simulink model "alternatesim1"  (Simulink 9.3)
settings: Solver=FixedStepAuto  StartTime=0.0  StopTime=7  RelTol=1e-3
libraries: neural x1
settings Model: Creator=Lenovo  LastModifiedBy=Lenovo
settings DataIOCC: SaveFormat=Dataset  SignalLoggingSaveFormat=Dataset  ReturnWorkspaceOutputs=on
settings OptimizationCC: LifeSpan=auto
settings DebuggingCC: UnderspecifiedInitializationDetection=Simplified  MergeDetectMultiDrivingBlocksExec=error  FcnCallInpInsideContextMsg=error  SFUnexpectedBacktrackingDiag=error  SFNoUnconditionalDefaultTransitionDiag=error  SFExecutionAtInitializationDiag=warning  ArithmeticOperatorsInVariantConditions=error
settings HardwareCC: ProdBitPerPointer=64  ProdBitPerSizeT=64  ProdBitPerPtrDiffT=64  ProdLargestAtomicFloat=Float  ProdIntDivRoundTo=Zero  ProdEndianess=LittleEndian  ProdWordSize=64  ProdHWDeviceType=Intel->x86-64 (Windows64)
settings ModelReferenceCC: PropagateSignalLabelsOutOfModel=on
settings SFSimCC: SimUseLocalCustomCode=on
settings RTWCC: RTWUseLocalCustomCode=on
settings CodeAppCC: StateflowObjectComments=off
settings GRTTargetCC: TargetLangStandard=C99 (ISO)  CombineOutputUpdateFcns=on  GRTInterface=off
settings ConfigComp: CovMetricSettings=dwe  CovHtmlReporting=off  CovSaveCumulativeToWorkspaceVar=off  CovSaveSingleToWorkspaceVar=off  CovExternalEMLEnable=on

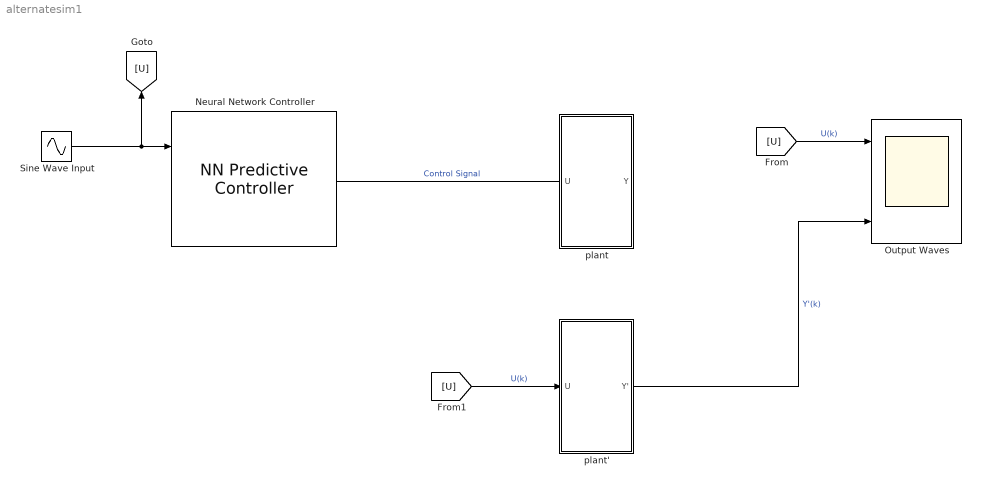
== system alternatesim1 ==
  Neural Network Controller : neural/Control Systems/NN Predictive Controller  epochs=150  minp=-1.4984328739291656873  maxp=1.4972411842840820384  mint=-0.49955219239929099517  maxt=1.4972411842840820384  Normalize=0  IW=[2.1565747230120617672 -0.3096984252732051246;-0.12313821449709881628 -0.1122642020318464634;-0.58041432517589952589 -0.21396504389264983659;0.19499335953396529364 -0.077631398333984871774;0.75410004063625590831 -0.16226526156567477877]  LW1_2=[0.5551207293764637285 0.018714294291257507069;-0.10132675699843593509 -0.027382341482495679841;-0.43309173846840326449 -0.0781007196607201859;-0.3314677820543142639 -0.032004154570293125159;-0.194985926119772085 -0.091076348073804089256]  LW2_1=[1.5809740000360821277 -1.0538130207537415028 -0.24233406046636835063 0.7751203522283688363 0.29703906315315625752]  B1=[-4.5237611134154054326;-0.05295680763842128963;1.2919589532592146153;0.17974555254224580669;-1.0663040710382076792]  B2=1.8293317221646907544  max_i_int=10  min_i_int=2  limit_output=0  max_output=Inf  min_output=-Inf  Use_Previous_Weights=1  N2=10  Nu=2  Ts=0.2  rho=0.05  alpha=0.001  csrchfun=csrchbac  maxiter=2  S1=5  Ni=2  Nj=2  sim_file=plant1  trainfun=trainbr  Use_validation=1  Use_Testing=0  max_i=1.5  min_i=-1.5  sam_training=10000
      settings: SourceProductName=MATLAB Runtime - Deep Learning Toolbox  SourceProductBaseCode=Missing
  Output Waves : Scope  NumInputPorts=3
  Sine Wave Input : Sin  Amplitude=0.8  Frequency=2  SampleTime=0.2
  plant : Subsystem
  plant' : Subsystem
  wires:
  ? -> Neural Network Controller/2, Output Waves/2  "Y(k)"
  Neural Network Controller/1 -> ?  "Control Signal"
  [U] -> Output Waves/1  "U(k)"
  [U] -> plant'/1(U)  "U(k)"
  plant'/1(Y') -> Output Waves/3  "Y'(k)"
  Sine Wave Input/1 -> [U], Neural Network Controller/1

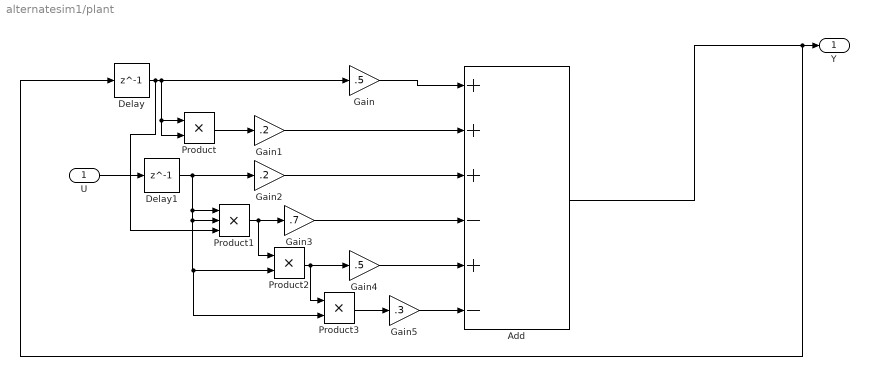
== system alternatesim1/plant ==
  U : Inport
  Add : Sum  Inputs=+++-+-
  Delay : Delay  DelayLength=1  InitialCondition=0
  Delay1 : Delay  DelayLength=1  InitialCondition=0
  Gain : Gain  Gain=.5
  Gain1 : Gain  Gain=.2
  Gain2 : Gain  Gain=.2
  Gain3 : Gain  Gain=.7
  Gain4 : Gain  Gain=.5
  Gain5 : Gain  Gain=.3
  Product : Product
  Product1 : Product  Inputs=3
  Product2 : Product
  Product3 : Product
  "Y " : Outport
  wires:
  Delay/1 -> Product1/3, Product/2, Product/1, Gain/1
  U/1 -> Delay1/1
  Gain5/1 -> Add/6
  Gain2/1 -> Add/3
  Product3/1 -> Gain5/1
  Add/1 -> Delay/1, "Y "/1
  Gain4/1 -> Add/5
  Product2/1 -> Product3/1, Gain4/1
  Delay1/1 -> Product3/2, Product2/2, Product1/2, Product1/1, Gain2/1
  Gain3/1 -> Add/4
  Product1/1 -> Product2/1, Gain3/1
  Gain/1 -> Add/1
  Product/1 -> Gain1/1
  Gain1/1 -> Add/2

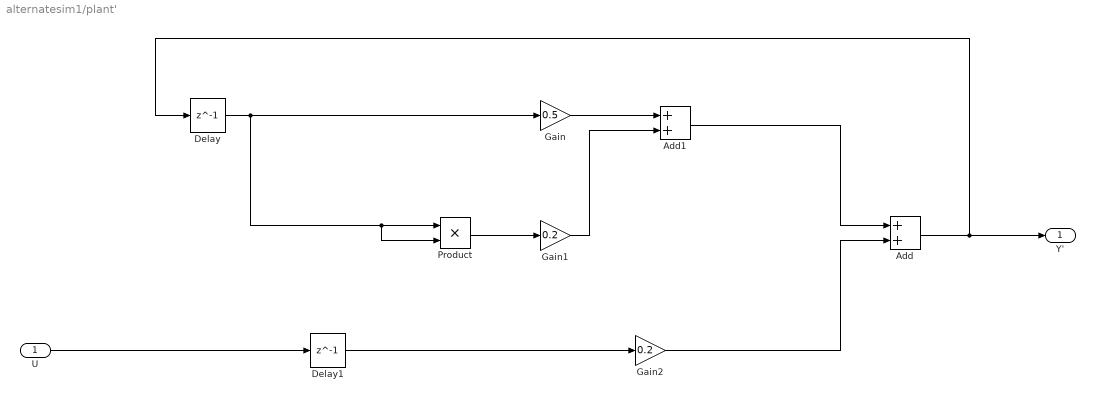
== system alternatesim1/plant' ==
  U : Inport
  Add : Sum
  Add1 : Sum
  Delay : Delay  DelayLength=1  InitialCondition=0  SampleTime=1e-4
  Delay1 : Delay  DelayLength=1  InitialCondition=0  SampleTime=1e-4
  Gain : Gain  Gain=0.5
  Gain1 : Gain  Gain=0.2
  Gain2 : Gain  Gain=0.2
  Product : Product
  Y' : Outport
  wires:
  Gain/1 -> Add1/1
  Delay/1 -> Product/2, Product/1, Gain/1
  Product/1 -> Gain1/1
  Gain2/1 -> Add/2
  Delay1/1 -> Gain2/1
  U/1 -> Delay1/1
  Add/1 -> Y'/1, Delay/1
  Gain1/1 -> Add1/2
  Add1/1 -> Add/1
